simulink model "reverse_emf"  (R2015b)
settings: Solver=VariableStepAuto  StartTime=0.0  StopTime=10  RelTol=1e-6
values from neighbouring files (symbols this model uses):
  Kt = .07329    (= 0.07329)    [Parameters.m]
  N = 4    [Parameters.m]
undefined symbols (not defined in the file or in its folder): phi_r, wc
libraries: fl_lib x5, pe_lib x4, nesl_utility x4, simulink x1
settings Model: Creator=Martin Andersen  LastModifiedBy=Martin Andersen

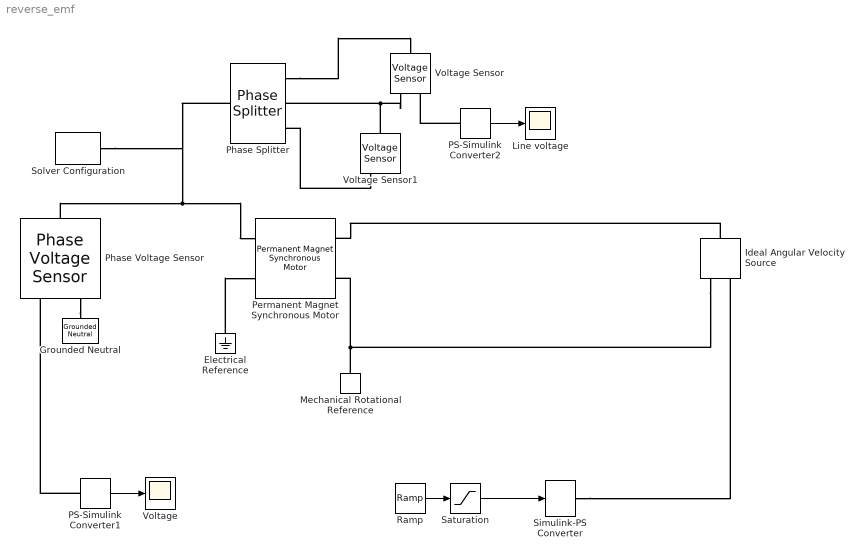
== system reverse_emf ==
  Electrical Reference : fl_lib/Electrical/Electrical Elements/Electrical Reference
  Grounded Neutral : pe_lib/Connections/Grounded Neutral
  Ideal Angular Velocity Source : fl_lib/Mechanical/Mechanical Sources/Ideal Angular Velocity Source
  Line voltage : Scope
  Mechanical Rotational Reference : fl_lib/Mechanical/Rotational Elements/Mechanical Rotational Reference
  PS-Simulink Converter1 : nesl_utility/PS-Simulink Converter  PhysicalDomain=network_engine_domain  SubClassName=ps_output  LeftPortType=input  RightPortType=output  PseudoPeriodic=off  Frequencies=[]  Unit=1  AffineConversion=off
  PS-Simulink Converter2 : nesl_utility/PS-Simulink Converter  PhysicalDomain=network_engine_domain  SubClassName=ps_output  LeftPortType=input  RightPortType=output  PseudoPeriodic=off  Frequencies=[]  Unit=1  AffineConversion=off
  Permanent Magnet Synchronous Motor : pe_lib/Machines/Permanent Magnet Rotor/Permanent Magnet Synchronous Motor  nPolePairs=N  pm_flux_linkage=Kt/N N*m/A  stator_param=1  Ld=.1 mH  Lq=.1 mH  L0=.1 mH  Ls=0.0002 H  Lm=0.00002 H  Ms=0.00002 H  Rs=R Ohm  initial_currents=[0, 0, 0] A  axes_param=2  angular_position0=phi_r/N rad  rotor_offset=- pi / 2 rad  shift_3ph=[nan, nan, nan] rad  sqrt2OverSqrt3=nan  oneOverSqrt2=nan  twoPiOver3=nan  Lmin=1e-9 H
  Phase Splitter : pe_lib/Connections/Phase Splitter
  Phase Voltage Sensor : pe_lib/Sensors/Phase Voltage Sensor
  Ramp : simulink/Sources/Ramp  slope=wc/5  start=0  X0=0
  Saturation : Saturate  UpperLimit=wc  LowerLimit=0
  Simulink-PS Converter : nesl_utility/Simulink-PS Converter  PhysicalDomain=network_engine_domain  SubClassName=ps_input  LeftPortType=input  RightPortType=output  PseudoPeriodic=off  Frequencies=[]  NoiseDistribution=none  NoiseParameters=[]  Unit=1  AffineConversion=off  InputFiltering=off  SimscapeFilterOrder=1  InputFilterTimeConstant=0.001  UdotUserProvided=1
  Solver Configuration : nesl_utility/Solver Configuration  PhysicalDomain=network_engine_domain  SubClassName=solver  LeftPortType=input  RightPortType=generic  Accelerate=off  Tones=[]  Harmonics=[]  SimulateNoise=off  Profile=off  UseLocalSampling=off  EnableSwitchedLinearOptims=on  FrequencyDomain=off  UseCCode=off  RelTol=0.001  AbsTol=1e-06  MinStep=1e-09  ToWorkspace=off  RevertToSquareIcSolve=off  NumHomotopyIterations=100  PhasorMode=off  PhasorModeNumHarmonics=1  DoDC=off  ResidualTolerance=1e-09  UseLocalSolver=off  LocalSolverChoice=NE_BACKWARD_EULER_ADVANCER  LocalSolverSampleTime=0.001  DoFixedCost=off  MaxNonlinIter=3  MaxModeIter=2  LinearAlgebra=Sparse  DelaysMemoryBudget=1024  AutomaticFiltering=on  FilteringTimeConstant=0.001
  Voltage : Scope
  Voltage Sensor : fl_lib/Electrical/Electrical Sensors/Voltage Sensor
  Voltage Sensor1 : fl_lib/Electrical/Electrical Sensors/Voltage Sensor
  wires:
  PS-Simulink Converter1/1 -> Voltage/1
  Ramp/1 -> Saturation/1
  Saturation/1 -> Simulink-PS Converter/1
  PS-Simulink Converter2/1 -> Line voltage/1
  connections:
  Phase Voltage Sensor/LConn1 -- Solver Configuration/RConn1 -- Phase Splitter/LConn1 -- Permanent Magnet Synchronous Motor/LConn1
  Electrical Reference/LConn1 -- Permanent Magnet Synchronous Motor/LConn2
  Phase Voltage Sensor/RConn2 -- Grounded Neutral/LConn1
  Ideal Angular Velocity Source/RConn2 -- Permanent Magnet Synchronous Motor/RConn2 -- Mechanical Rotational Reference/LConn1
  PS-Simulink Converter1/LConn1 -- Phase Voltage Sensor/RConn1
  Ideal Angular Velocity Source/LConn1 -- Permanent Magnet Synchronous Motor/RConn1
  Simulink-PS Converter/RConn1 -- Ideal Angular Velocity Source/RConn1
  Voltage Sensor/RConn2 -- Phase Splitter/RConn2 -- Voltage Sensor1/LConn1
  Phase Splitter/RConn1 -- Voltage Sensor/LConn1
  PS-Simulink Converter2/LConn1 -- Voltage Sensor/RConn1
  Voltage Sensor1/RConn2 -- Phase Splitter/RConn3
